simulink model "sampleModel1897_5"  (R2023a)
settings: Solver=VariableStepAuto  StartTime=0.0  StopTime=10.0  RelTol=1e-3
libraries: hdlsllib x4, simulink x3
settings Model: Creator=user1  LastModifiedBy=user1

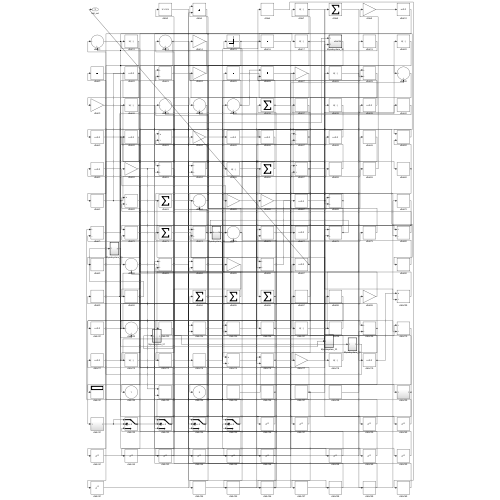
[thumbnail: Simulink's stored preview of the top-level diagram]
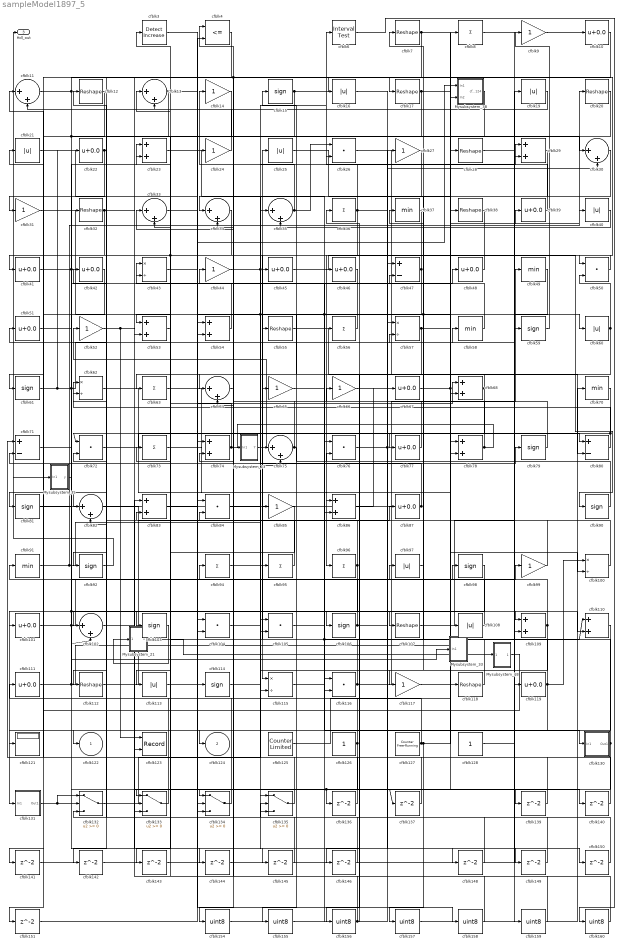
== system sampleModel1897_5 ==
  Mysubsystem_13 : Subsystem  TreatAsAtomicUnit=on  RTWFcnName=Mysubsystem_13
      settings: RTWFcnNameOpts=User specified  RTWFileNameOpts=Use function name
  Mysubsystem_18 : Subsystem  TreatAsAtomicUnit=on  RTWFcnName=Mysubsystem_18
      settings: RTWFcnNameOpts=User specified  RTWFileNameOpts=Use function name
  Mysubsystem_21 : Subsystem  TreatAsAtomicUnit=on  RTWFcnName=Mysubsystem_21
      settings: RTWFcnNameOpts=User specified  RTWFileNameOpts=Use function name
  Mysubsystem_33 : Subsystem  TreatAsAtomicUnit=on  RTWFcnName=Mysubsystem_33
      settings: RTWFcnNameOpts=User specified  RTWFileNameOpts=Use function name
  Mysubsystem_35 : Subsystem  TreatAsAtomicUnit=on  RTWFcnName=Mysubsystem_35
      settings: RTWFcnNameOpts=User specified  RTWFileNameOpts=Use function name
  Mysubsystem_38 : Subsystem  TreatAsAtomicUnit=on  RTWFcnName=Mysubsystem_38
      settings: RTWFcnNameOpts=User specified  RTWFileNameOpts=Use function name
  cfblk{10,22,39,41..42,45..46,48,51,67,77,87,101,111,119} (15 alike) : Bias  Bias=0.0  SaturateOnIntegerOverflow=off
  cfblk{43,57,62,100,115} (5 alike) : Product  Inputs=*/  OutDataTypeStr=uint8  RndMeth=Zero  SaturateOnIntegerOverflow=on
  cfblk{11,13,30,33..35,64,75,82,102} (10 alike) : Sum  Inputs=|++  OutDataTypeStr=uint8
  cfblk{15,59,61,79,81,90,92,98,103,106,114} (11 alike) : Signum
  cfblk{26,50,72,76,84,104..105,116} (8 alike) : DotProduct  OutDataTypeStr=uint8
  cfblk{7,12,17,20,28,32,38,55,107,112,118} (11 alike) : Reshape
  cfblk{16,19,21,25,40,60,97,108,113} (9 alike) : Abs  OutDataTypeStr=uint8  SaturateOnIntegerOverflow=off
  cfblk{23,29,53..54,68,74,78,83,86,109..110} (11 alike) : Sum  OutDataTypeStr=uint8
  cfblk{9,14,24,27,31,44,52,65..66,85,99,117} (12 alike) : Gain  OutDataTypeStr=uint8
  cfblk121 : Display
  cfblk123 : Record  FileSettingsInternal="{\"entries\":[{\"content\":{\"excelSettings\":{\"content\":{},\"type\":\"Streamout.ExcelSettings\"}},\"type\":\"Streamout.FileSettingStorage\",\"uuid\":\"\"}],\"packageUris\":[\"http:\\/\\/schema.mathworks.com\\/mf0\\/streamout_blocks\\/R2020a\"],\"version\":\"1.0\"}"  Layout=[1 1]  SignalsInternal="{\"entries\":[{\"content\":{\"signals\":[{\"content\":{\"blockPath\":[],\"dimensions\":[1],\"domain\":\"\",\"lineColor\":\"#a2142f\",\"plots\":[1],\"port\":1,\"signalID\":49652,\"signalName\":\"cfblk52\"},\"type\":\"RecordBlkView.Signal\",\"uuid\":\"\"},{\"content\":{\"blockPath\":[],\"dimensions\":[1],\"domain\":\"\",\"lineColor\":\"#139fff\",\"plots\":[1],\"port\":2,\"signalID\":49655,\"signalName\":\"cfblk20\"},\"type\":\"RecordBlkView.Signal\",\"uuid\":\"\"}]},\"type\":\"RecordBlkView.InputSignals\",\"uuid\":\"\"}],\"packageUris\":[\"http:\\/\\/schema.mathworks.com\\/mf0\\/streamout_blocks\\/R2020a\"],\"version\":\"1.0\"}"  VisualizationBindings="{\"xyplotplugin\":{\"info\":[{\"series\":[{\"bindingParametersList\":[{\"parameter\":\"X-Axis\",\"signalID\":49652,\"signalName\":\"cfblk52\"},{\"parameter\":\"Y-Axis\",\"signalID\":49655,\"signalName\":\"cfblk20\"}],\"seriesID\":55499}],\"subplotID\":1}]}}"  CompatibilityTag=XY  st=-1
  cfblk125 : hdlsllib/Sources/Counter Limited  uplimit=7  tsamp=-1
  cfblk126 : Constant  OutDataTypeStr=uint8  SampleTime=-1
  cfblk127 : hdlsllib/Sources/Counter Free-Running  NumBits=16  tsamp=-1
  cfblk128 : Constant  OutDataTypeStr=uint8  SampleTime=-1
  cfblk130 : Subsystem
      settings: LibrarySourceBlock=|
      | hdlsllib/Ports &
      | Subsystems/Subsystem
  cfblk131 : Subsystem
      settings: LibrarySourceBlock=|
      | hdlsllib/Ports &
      | Subsystems/Subsystem
  cfblk{132..135} (4 alike) : Switch  OutDataTypeStr=uint8  SaturateOnIntegerOverflow=off  InputSameDT=off
  cfblk{136..137,139..146,148..151} (14 alike) : Delay  SampleTime=1
  cfblk{154..160} (7 alike) : DataTypeConversion  OutDataTypeStr=uint8  SaturateOnIntegerOverflow=off  RndMeth=Floor
  cfblk3 : simulink/Logic and Bit Operations/Detect Increase  vinit=0.0  OutDataTypeStr=uint8
      settings: LibrarySourceBlock=|
      | hdlsllib/Logic and Bit
      | Operations/Detect
      | Increase
  cfblk{8,36,56,63,73,94..96} (8 alike) : Sum  Inputs=+  OutDataTypeStr=uint8
  cfblk{37,49,58,70,91} (5 alike) : MinMax  OutDataTypeStr=uint8
  cfblk4 : RelationalOperator  Operator=<=  OutDataTypeStr=boolean  InputSameDT=off
  cfblk47 : Sum  Inputs=+-  OutDataTypeStr=uint8
  cfblk6 : hdlsllib/Logic and Bit Operations/Interval Test  IntervalClosedRight=on  uplimit=0.5  IntervalClosedLeft=on  lowlimit=-0.5  OutDataTypeStr=uint8
  cfblk71 : Sum  Inputs=+-  OutDataTypeStr=uint8
  cfblk80 : Sum  Inputs=+-  OutDataTypeStr=uint8
  cfblk122 : Outport  OutDataTypeStr=uint8  VectorParamsAs1DForOutWhenUnconnected=off
  cfblk124 : Outport  Port=2  OutDataTypeStr=uint8  VectorParamsAs1DForOutWhenUnconnected=off
  Hdl_out : Outport  Port=3  OutDataTypeStr=uint8
  wires:
  cfblk86/1 -> cfblk67/1
  cfblk116/1 -> cfblk49/1, cfblk73/1
  cfblk52/1 -> cfblk123/1, cfblk57/2
  cfblk35/1 -> cfblk14/1, cfblk26/1
  cfblk80/1 -> cfblk72/1, cfblk62/2
  cfblk91/1 -> cfblk20/1, cfblk75/2
  cfblk100/1 -> cfblk51/1
  cfblk130/1(Out1) -> cfblk25/1, cfblk134/2
  cfblk15/1 -> cfblk50/1, cfblk134/1
  cfblk45/1 -> cfblk90/1
  cfblk39/1 -> cfblk6/1
  cfblk38/1 -> cfblk115/1
  cfblk73/1 -> cfblk135/1
  cfblk132/1 -> cfblk95/1
  cfblk49/1 -> cfblk107/1, cfblk104/2
  cfblk36/1 -> cfblk96/1, cfblk26/2, cfblk30/2
  cfblk72/1 -> cfblk77/1
  cfblk99/1 -> cfblk75/1
  cfblk48/1 -> cfblk46/1
  cfblk10/1 -> cfblk34/1, cfblk53/2
  cfblk79/1 -> cfblk66/1
  cfblk31/1 -> cfblk114/1
  cfblk119/1 -> cfblk7/1, cfblk100/1, cfblk134/3
  cfblk30/1 -> cfblk115/2
  cfblk82/1 -> cfblk87/1
  cfblk58/1 -> cfblk44/1
  cfblk133/1 -> cfblk12/1
  cfblk76/1 -> cfblk58/1, cfblk149/1
  cfblk23/1 -> cfblk116/2
  cfblk66/1 -> cfblk80/1
  cfblk32/1 -> cfblk61/1, cfblk145/1
  cfblk26/1 -> cfblk119/1
  cfblk77/1 -> cfblk43/1
  cfblk112/1 -> cfblk85/1
  cfblk20/1 -> cfblk123/2
  cfblk47/1 -> cfblk86/2, cfblk65/1, cfblk45/1
  cfblk60/1 -> cfblk50/2, cfblk146/1
  cfblk57/1 -> Mysubsystem_38/2(In2), cfblk64/1
  cfblk7/1 -> cfblk38/1, cfblk151/1
  cfblk62/1 -> cfblk118/1
  cfblk55/1 -> cfblk80/2
  cfblk61/1 -> cfblk59/1, cfblk144/1, cfblk22/1
  cfblk84/1 -> cfblk16/1
  cfblk34/1 -> cfblk133/1, cfblk142/1
  cfblk96/1 -> cfblk131/1(In1), cfblk62/1
  cfblk101/1 -> cfblk99/1, cfblk97/1
  cfblk113/1 -> cfblk68/1
  cfblk67/1 -> cfblk39/1, cfblk140/1
  cfblk126/1 -> cfblk94/1, cfblk133/3
  cfblk118/1 -> cfblk43/2
  cfblk65/1 -> cfblk130/1(In1)
  cfblk12/1 -> cfblk81/1
  cfblk37/1 -> cfblk102/1
  cfblk4/1 -> cfblk82/1
  cfblk24/1 -> cfblk11/2
  cfblk85/1 -> cfblk113/1
  cfblk75/1 -> cfblk33/1, cfblk155/1
  cfblk108/1 -> cfblk21/1
  cfblk74/1 -> cfblk109/1, cfblk33/2
  cfblk56/1 -> cfblk55/1
  cfblk71/1 -> cfblk48/1
  cfblk114/1 -> cfblk105/1
  cfblk59/1 -> cfblk9/1
  cfblk97/1 -> cfblk37/1
  cfblk131/1(Out1) -> cfblk132/1, cfblk132/2
  cfblk111/1 -> cfblk32/1, cfblk8/1
  cfblk94/1 -> cfblk35/1
  cfblk110/1 -> cfblk121/1
  cfblk107/1 -> cfblk19/1
  cfblk29/1 -> cfblk117/1
  cfblk78/1 -> Mysubsystem_13/1(In1), cfblk34/2
  cfblk51/1 -> cfblk23/1
  cfblk134/1 -> cfblk111/1
  cfblk17/1 -> cfblk103/1, cfblk100/2
  cfblk95/1 -> cfblk24/1
  cfblk19/1 -> cfblk13/2
  cfblk22/1 -> cfblk31/1, cfblk92/1
  cfblk14/1 -> cfblk53/1
  cfblk102/1 -> cfblk136/1, cfblk137/1
  cfblk109/1 -> cfblk36/1, cfblk135/3
  cfblk128/1 -> cfblk40/1
  cfblk135/1 -> cfblk91/1
  cfblk127/1 -> cfblk28/1, cfblk157/1, cfblk42/1
  cfblk40/1 -> cfblk35/2
  cfblk11/1 -> cfblk133/2, cfblk29/2, cfblk17/1
  cfblk46/1 -> cfblk105/2, cfblk54/2
  cfblk44/1 -> cfblk29/1, cfblk148/1
  cfblk70/1 -> cfblk156/1
  cfblk63/1 -> cfblk86/1
  cfblk3/1 -> cfblk74/1
  cfblk87/1 -> cfblk71/2, Hdl_out/1
  cfblk9/1 -> cfblk10/1
  cfblk8/1 -> cfblk60/1
  cfblk117/1 -> cfblk78/1
  cfblk104/1 -> cfblk79/1
  cfblk25/1 -> cfblk108/1
  cfblk81/1 -> cfblk102/2, cfblk110/2
  cfblk125/1 -> cfblk78/2
  cfblk41/1 -> cfblk68/2, cfblk106/1
  cfblk105/1 -> cfblk56/1
  cfblk13/1 -> cfblk30/1, cfblk112/1
  cfblk90/1 -> cfblk15/1
  cfblk68/1 -> cfblk122/1, cfblk63/1
  cfblk21/1 -> cfblk104/1
  cfblk106/1 -> cfblk98/1, cfblk72/2
  cfblk50/1 -> cfblk41/1
  cfblk54/1 -> cfblk3/1
  cfblk64/1 -> cfblk4/1
  cfblk42/1 -> cfblk101/1
  cfblk115/1 -> cfblk110/1, cfblk47/2
  cfblk136/1 -> cfblk71/1
  cfblk137/1 -> cfblk74/2
  cfblk16/1 -> cfblk139/1
  cfblk139/1 -> cfblk54/1
  cfblk140/1 -> cfblk47/1
  cfblk98/1 -> cfblk141/1
  cfblk141/1 -> cfblk116/1
  cfblk142/1 -> cfblk57/1
  cfblk53/1 -> cfblk143/1
  cfblk143/1 -> cfblk13/1
  cfblk144/1 -> cfblk109/2
  cfblk145/1 -> cfblk132/3
  cfblk146/1 -> cfblk64/2
  cfblk148/1 -> cfblk82/2
  cfblk149/1 -> cfblk23/2
  cfblk33/1 -> cfblk150/1
  cfblk150/1 -> cfblk135/2
  cfblk151/1 -> cfblk4/2
  cfblk27/1 -> cfblk154/1
  cfblk154/1 -> cfblk76/1
  cfblk155/1 -> cfblk27/1
  cfblk156/1 -> cfblk84/2, cfblk76/2
  cfblk157/1 -> cfblk70/1
  cfblk83/1 -> cfblk158/1
  cfblk158/1 -> cfblk84/1
  cfblk28/1 -> cfblk159/1
  cfblk159/1 -> cfblk83/1
  cfblk6/1 -> cfblk160/1
  cfblk160/1 -> cfblk83/2
  Mysubsystem_13/1(Y) -> cfblk52/1
  Mysubsystem_18/1(Out1) -> cfblk11/1
  cfblk103/1 -> Mysubsystem_21/1(In1)
  Mysubsystem_21/1(Out1) -> Mysubsystem_18/1(In1)
  cfblk92/1 -> Mysubsystem_35/1(In1)
  Mysubsystem_35/1(y) -> Mysubsystem_33/1(In1)
  cfblk43/1 -> Mysubsystem_38/1(In1)
  Mysubsystem_38/1(cfblk124) -> cfblk124/1

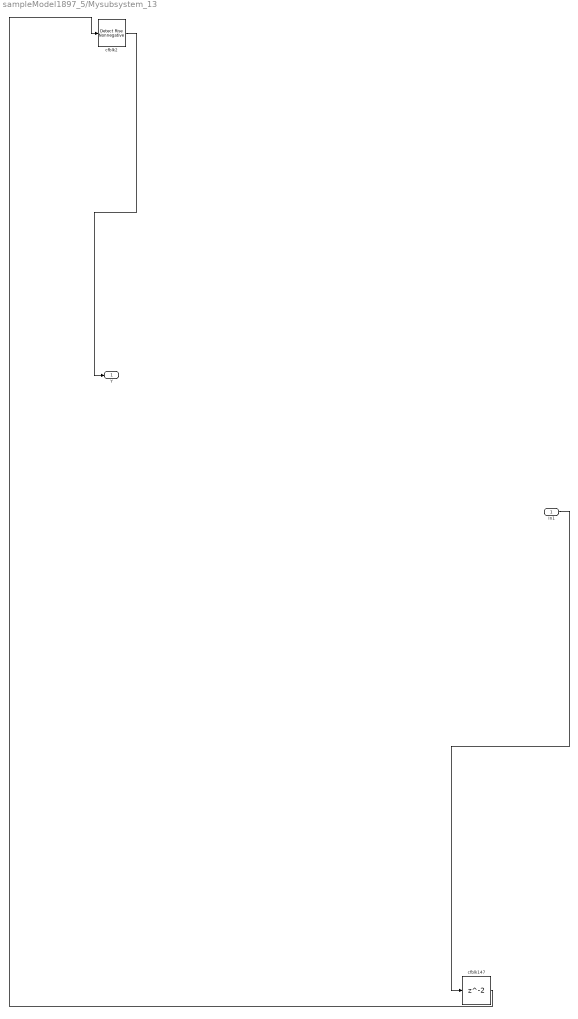
== system sampleModel1897_5/Mysubsystem_13 ==
  In1 : Inport
  cfblk147 : Delay  SampleTime=1
  cfblk2 : hdlsllib/Logic and Bit Operations/Detect Rise Nonnegative  vinit=0  OutDataTypeStr=boolean
  Y : Outport
  wires:
  cfblk147/1 -> cfblk2/1
  cfblk2/1 -> Y/1
  In1/1 -> cfblk147/1

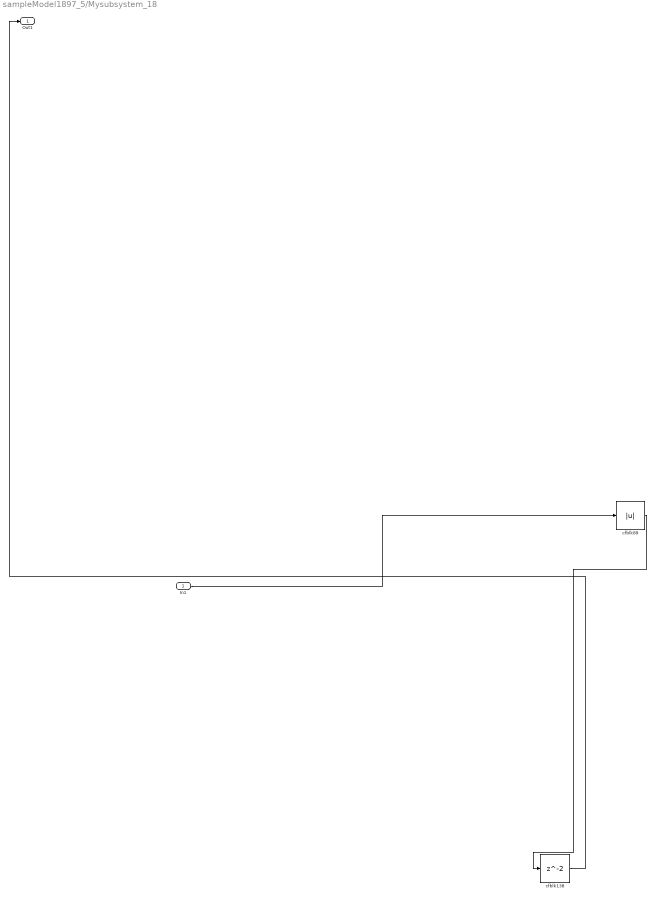
== system sampleModel1897_5/Mysubsystem_18 ==
  In1 : Inport
  cfblk138 : Delay  SampleTime=1
  cfblk89 : Abs  SaturateOnIntegerOverflow=off
  Out1 : Outport
  wires:
  cfblk89/1 -> cfblk138/1
  cfblk138/1 -> Out1/1
  In1/1 -> cfblk89/1

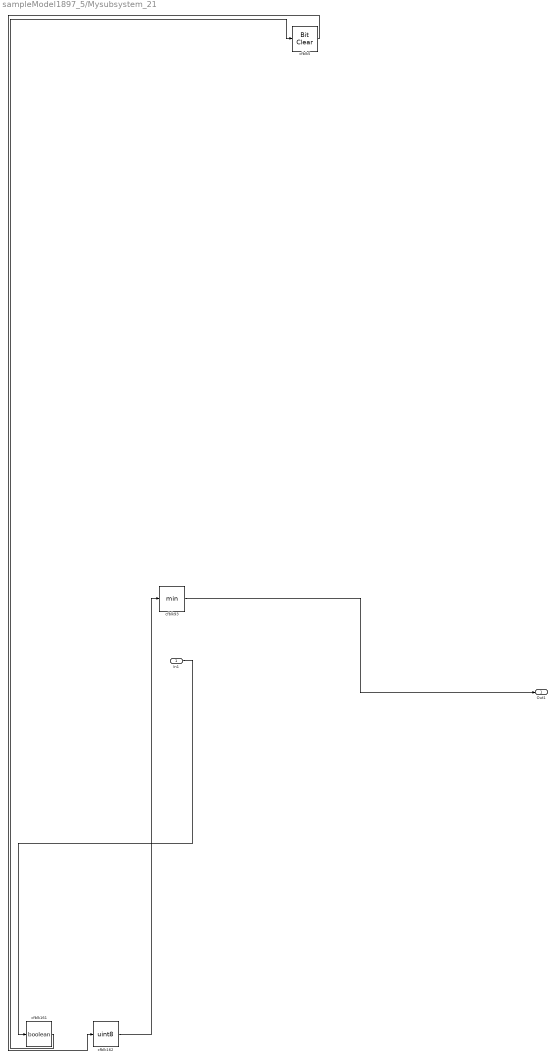
== system sampleModel1897_5/Mysubsystem_21 ==
  In1 : Inport
  cfblk161 : DataTypeConversion  OutDataTypeStr=boolean  SaturateOnIntegerOverflow=off  RndMeth=Floor
  cfblk162 : DataTypeConversion  OutDataTypeStr=uint8  SaturateOnIntegerOverflow=off  RndMeth=Floor
  cfblk5 : simulink/Logic and Bit Operations/Bit Clear  iBit=0
      settings: LibrarySourceBlock=|
      | hdlsllib/Logic and Bit
      | Operations/Bit Clear
  cfblk93 : MinMax
  Out1 : Outport
  wires:
  cfblk93/1 -> Out1/1
  In1/1 -> cfblk161/1
  cfblk5/1 -> cfblk162/1
  cfblk161/1 -> cfblk5/1
  cfblk162/1 -> cfblk93/1

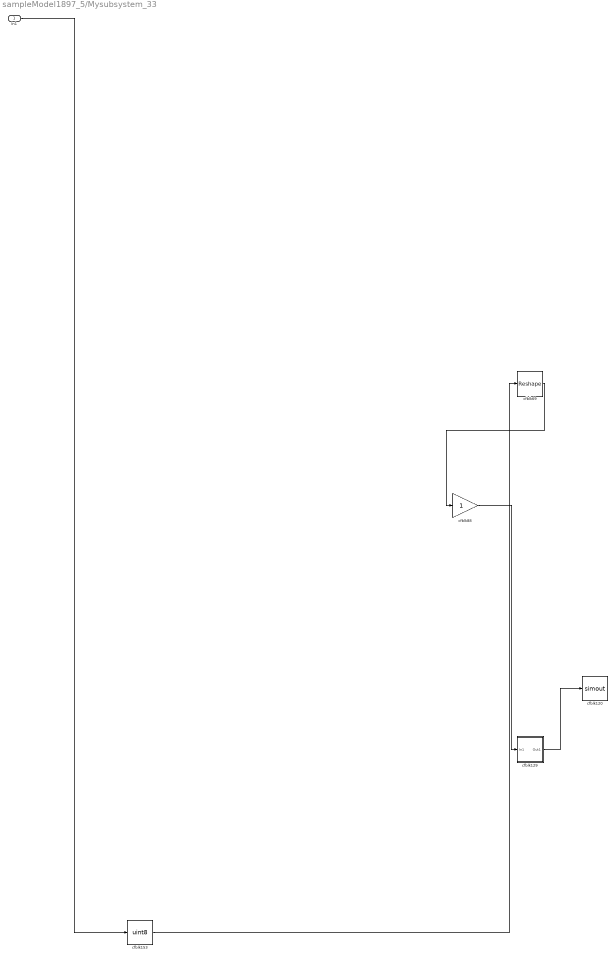
== system sampleModel1897_5/Mysubsystem_33 ==
  In1 : Inport
  cfblk120 : ToWorkspace  VariableName=simout  SaveFormat=Timeseries  SampleTime=-1
  cfblk129 : Subsystem
      settings: LibrarySourceBlock=|
      | hdlsllib/Ports &
      | Subsystems/Subsystem
  cfblk153 : DataTypeConversion  OutDataTypeStr=uint8  SaturateOnIntegerOverflow=off  RndMeth=Floor
  cfblk69 : Reshape
  cfblk88 : Gain
  wires:
  cfblk153/1 -> cfblk69/1
  cfblk88/1 -> cfblk129/1(In1)
  cfblk69/1 -> cfblk88/1
  In1/1 -> cfblk153/1
  cfblk129/1(Out1) -> cfblk120/1

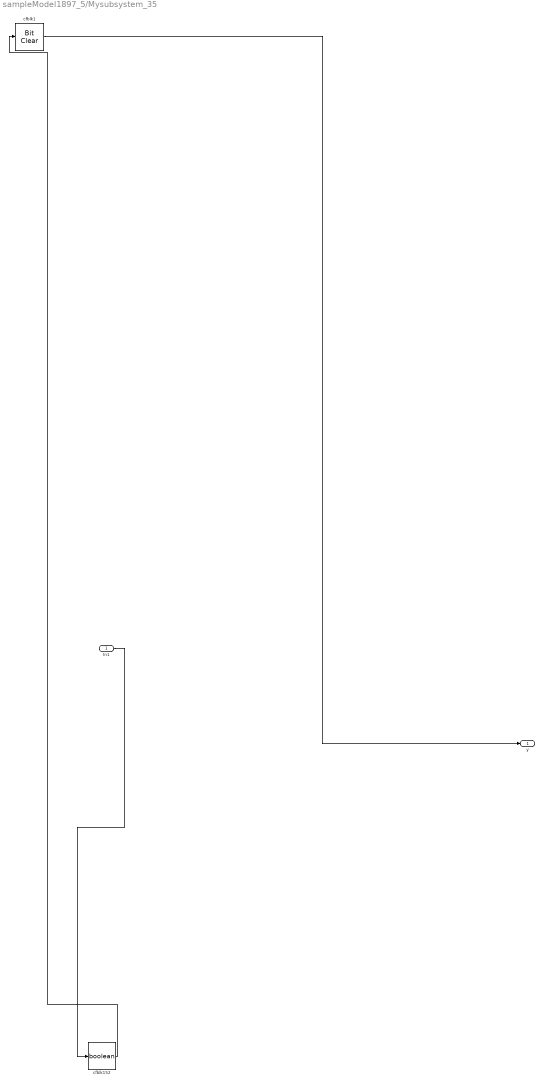
== system sampleModel1897_5/Mysubsystem_35 ==
  In1 : Inport
  cfblk1 : simulink/Logic and Bit Operations/Bit Clear  iBit=0
      settings: LibrarySourceBlock=|
      | hdlsllib/Logic and Bit
      | Operations/Bit Clear
  cfblk152 : DataTypeConversion  OutDataTypeStr=boolean  SaturateOnIntegerOverflow=off  RndMeth=Floor
  y : Outport
  wires:
  cfblk152/1 -> cfblk1/1
  In1/1 -> cfblk152/1
  cfblk1/1 -> y/1

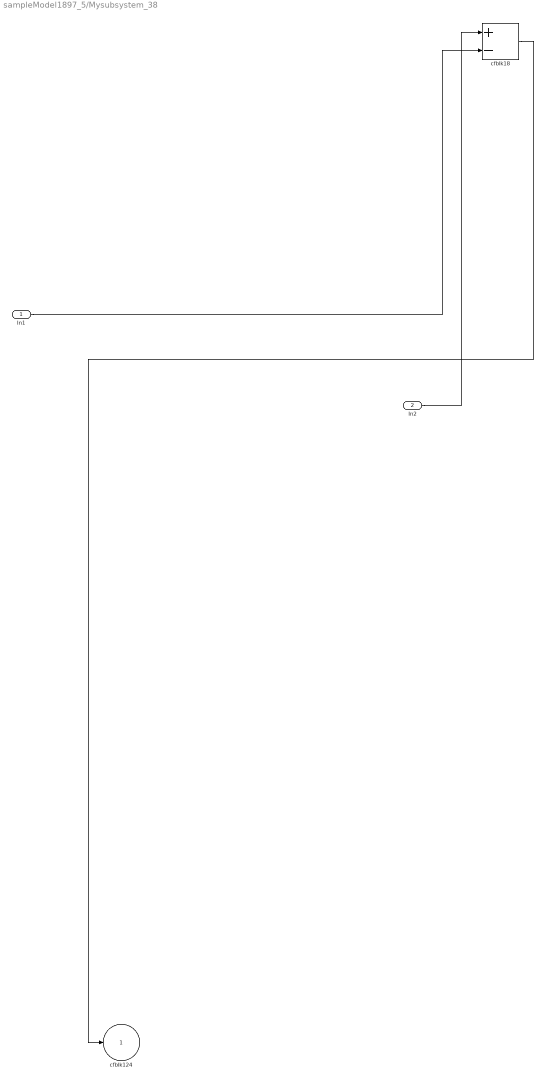
== system sampleModel1897_5/Mysubsystem_38 ==
  In1 : Inport
  In2 : Inport  Port=2
  cfblk18 : Sum  Inputs=+-
  cfblk124 : Outport  VectorParamsAs1DForOutWhenUnconnected=off
  wires:
  cfblk18/1 -> cfblk124/1
  In1/1 -> cfblk18/2
  In2/1 -> cfblk18/1

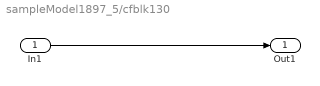
== system sampleModel1897_5/cfblk130 ==
  In1 : Inport
  Out1 : Outport
  wires:
  In1/1 -> Out1/1

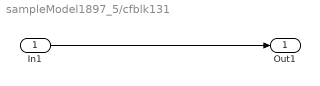
== system sampleModel1897_5/cfblk131 ==
  In1 : Inport
  Out1 : Outport
  wires:
  In1/1 -> Out1/1

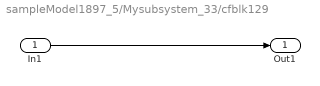
== system sampleModel1897_5/Mysubsystem_33/cfblk129 ==
  In1 : Inport
  Out1 : Outport
  wires:
  In1/1 -> Out1/1
